simulink model "RGB"  (R2018b)
settings: Solver=FixedStepAuto  StartTime=0.0  StopTime=SIM_TIME  FixedStep=0.01  RelTol=1e-3  EnableMultiTasking=on
values from neighbouring files (symbols this model uses):
  PWM_AMPLITUDE = 125    [Parameters.m]
  SINE_SAMPLE_TIME = 0.01    [Parameters.m]
libraries: arduinolib x3
settings Model: ExtModeTrigDuration=2  Creator=alessandrosebastianelli  LastModifiedBy=alessandrosebastianelli
settings OptimizationCC: EnhancedBackFolding=on  PassReuseOutputArgsAs=Individual arguments  MaxStackSize=64  OptimizeBlockOrder=speed  DifferentSizesBufferReuse=on  OptimizationCustomize=off
settings DebuggingCC: ParameterTunabilityLossMsg=error
settings HardwareCC: ProdBitPerInt=16  ProdBitPerPointer=16  ProdBitPerSizeT=16  ProdBitPerPtrDiffT=16  ProdLargestAtomicFloat=None  ProdWordSize=8  ProdHWDeviceType=Atmel->AVR  UseEmbeddedCoderFeatures=off  UseSimulinkCoderFeatures=off
settings SFSimCC: MATLABDynamicMemAlloc=off
settings RTWCC: SystemTargetFile=ert.tlc  HardwareBoard=Arduino Mega 2560  TemplateMakefile=ert_default_tmf  GenerateReport=on  Toolchain=Arduino AVR  BuildConfiguration=Faster Runs  IncludeHyperlinkInReport=on  LaunchReport=on  GenerateTraceInfo=on  GenerateTraceReport=on  GenerateTraceReportSl=on  GenerateTraceReportSf=on  GenerateTraceReportEml=on
settings CodeAppCC: ForceParamTrailComments=on  IgnoreCustomStorageClasses=off  OperatorAnnotations=on  SimulinkDataObjDesc=on  SFDataObjDesc=on  InsertBlockDesc=on
settings ERTTargetCC: SupportContinuousTime=on  SupportNonInlinedSFcns=on  SupportVariableSizeSignals=on

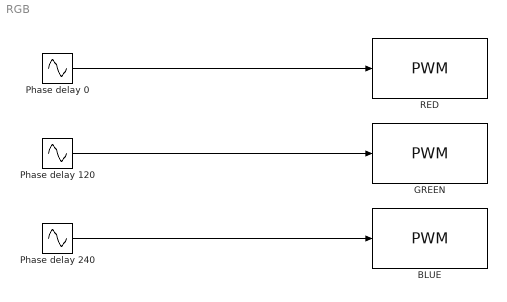
== system RGB ==
  BLUE : arduinolib/PWM  pinNumber=BLUE_PIN  EnableInputFrequency=off  InitialFrequency=2000  InitialDutyCycle=0  NotificationType=None  blockPlatform=arduino
  GREEN : arduinolib/PWM  pinNumber=GREEN_PIN  EnableInputFrequency=off  InitialFrequency=2000  InitialDutyCycle=0  NotificationType=None  blockPlatform=arduino
  Phase delay 0 : Sin  SineType=Sample based  Amplitude=PWM_AMPLITUDE  Bias=PWM_AMPLITUDE  Samples=SAMPLE_PER_PERIOD  SampleTime=SINE_SAMPLE_TIME  Offset=PHASE_DELAY_R
  Phase delay 120 : Sin  SineType=Sample based  Amplitude=PWM_AMPLITUDE  Bias=PWM_AMPLITUDE  Samples=SAMPLE_PER_PERIOD  SampleTime=SINE_SAMPLE_TIME  Offset=PHASE_DELAY_G
  Phase delay 240 : Sin  SineType=Sample based  Amplitude=PWM_AMPLITUDE  Bias=PWM_AMPLITUDE  Samples=SAMPLE_PER_PERIOD  SampleTime=SINE_SAMPLE_TIME  Offset=PHASE_DELAY_B
  RED : arduinolib/PWM  pinNumber=RED_PIN  EnableInputFrequency=off  InitialFrequency=2000  InitialDutyCycle=0  NotificationType=None  blockPlatform=arduino
  wires:
  Phase delay 0/1 -> RED/1
  Phase delay 120/1 -> GREEN/1
  Phase delay 240/1 -> BLUE/1
